simulink model "sim_controller"  (R2017a)
settings: Solver=ode45  StartTime=0.0  StopTime=inf  RelTol=1e-3  EnableMultiTasking=on
undefined symbols (not defined in the file): CR, serial
libraries: instrumentlib x3
settings Model: Creator=sagar  LastModifiedBy=ismaelm
settings DataIOCC: LimitDataPoints=on  SaveFormat=Array
settings OptimizationCC: LifeSpan=inf
settings DebuggingCC: SolverPrmCheckMsg=warning  SFUnexpectedBacktrackingDiag=warning  SFNoUnconditionalDefaultTransitionDiag=warning  SFExecutionAtInitializationDiag=none
settings HardwareCC: ProdBitPerPointer=32  ProdBitPerSizeT=32  ProdBitPerPtrDiffT=32  ProdLargestAtomicFloat=None  ProdIntDivRoundTo=Undefined  ProdEndianess=Unspecified  ProdWordSize=32  ProdHWDeviceType=32-bit Generic
settings ModelReferenceCC: PropagateSignalLabelsOutOfModel=off
settings GRTTargetCC: TargetLangStandard=C89/C90 (ANSI)  GeneratePreprocessorConditionals=Disable all
settings ConfigComp: CovMetricSettings=dw  CovHtmlReporting=on  CovSaveCumulativeToWorkspaceVar=on  CovSaveSingleToWorkspaceVar=on  CovExternalEMLEnable=off  CovSFcnEnable=off

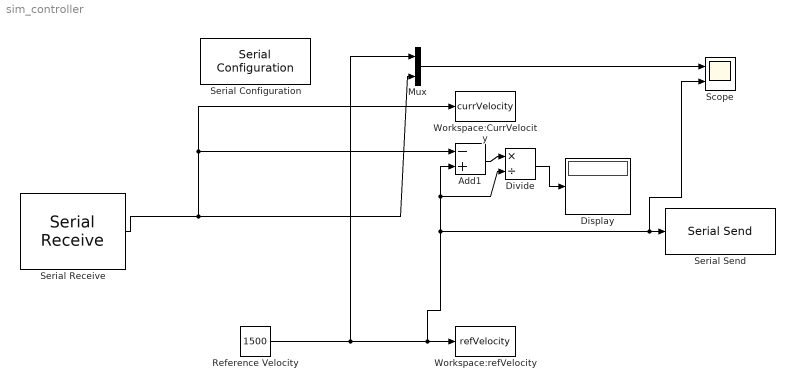
== system sim_controller ==
  Add1 : Sum  Inputs=-+
  Display : Display
  Divide : Product  Inputs=*/
  Mux : Mux  Inputs=2
  Reference Velocity : Constant  Value=1500  OutDataTypeStr=single  SampleTime=0.1
  Scope : Scope  NumInputPorts=2
  Serial Configuration : instrumentlib/Serial Configuration  Priority=-200000  ComPortMenu=COM12  ComPort=COM12  ObjConstructor=serial('COM12');  BaudRate=115200  DataBits=8  Parity=none  StopBits=1  FlowControl=none  Timeout=10  ByteOrder=LittleEndian
  Serial Receive : instrumentlib/Serial Receive  ComPortMenu=COM12  ComPort=COM12  ObjConstructor=serial('COM12');  Terminator=<none>  DataSize="[1  1]"  DataType=single  EnableBlockingMode=on  ActionDataUnavailable=Output last received value  CustomValue=0  SampleTime=0.1
  Serial Send : instrumentlib/Serial Send  ComPortMenu=COM12  ComPort=COM12  ObjConstructor=serial('COM12');  Terminator=CR ('\r')  EnableBlockingMode=on
  Workspace:CurrVelocity : ToWorkspace  VariableName=currVelocity  SaveFormat=Timeseries  SampleTime=-1
  Workspace:refVelocity : ToWorkspace  VariableName=refVelocity  SaveFormat=Timeseries  SampleTime=-1
  wires:
  Reference Velocity/1 -> Mux/1, Scope/2, Serial Send/1, Divide/2, Add1/2, Workspace:refVelocity/1
  Mux/1 -> Scope/1
  Add1/1 -> Divide/1
  Divide/1 -> Display/1
  Serial Receive/1 -> Mux/2, Workspace:CurrVelocity/1, Add1/1
